simulink model "exp6"  (R2025b)
settings: Solver=VariableStepAuto  StartTime=0.0  StopTime=10.0  RelTol=1e-3
settings Model: Creator=SUBHASH  LastModifiedBy=SUBHASH

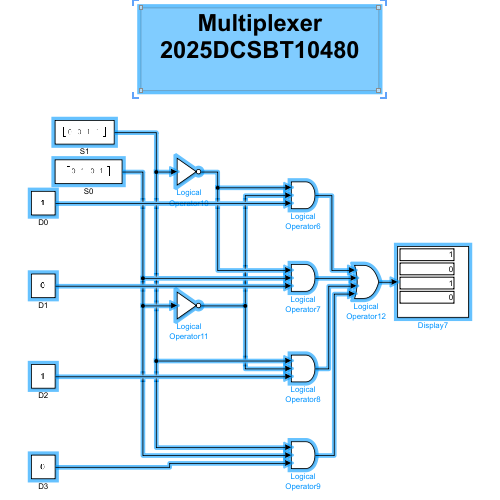
[thumbnail: Simulink's stored preview of the top-level diagram]
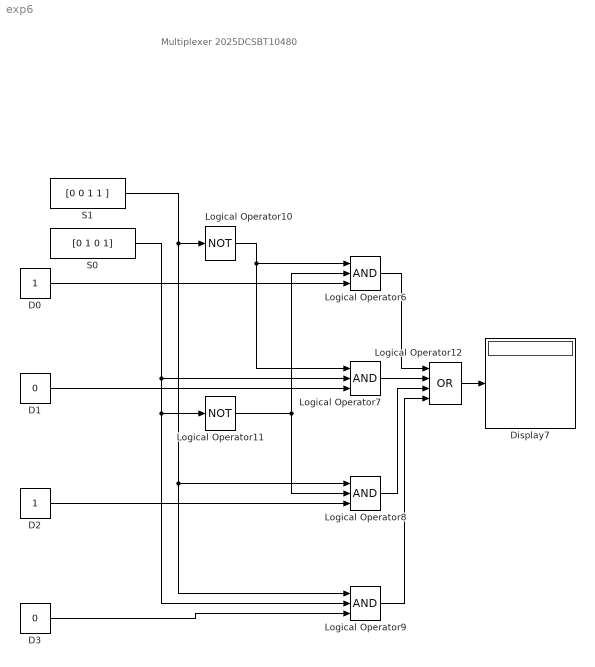
== system exp6 ==
  note: Multiplexer
      | 2025DCSBT10480
  D0 : Constant
  D1 : Constant  Value=0
  D2 : Constant
  D3 : Constant  Value=0
  Display7 : Display
  Logical Operator10 : Logic  Operator=NOT  IconShape=distinctive  AllPortsSameDT=off  OutDataTypeStr=boolean
  Logical Operator11 : Logic  Operator=NOT  IconShape=distinctive  AllPortsSameDT=off  OutDataTypeStr=boolean
  Logical Operator12 : Logic  Operator=OR  Inputs=4  IconShape=distinctive  AllPortsSameDT=off  OutDataTypeStr=boolean
  Logical Operator{6..9} (4 alike) : Logic  Inputs=3  IconShape=distinctive  AllPortsSameDT=off  OutDataTypeStr=boolean
  S0 : Constant  Value=[0 1 0 1]
  S1 : Constant  Value=[0 0 1 1 ]
  wires:
  D2/1 -> Logical Operator8/3
  D0/1 -> Logical Operator6/3
  Logical Operator10/1 -> Logical Operator7/1, Logical Operator6/1
  Logical Operator12/1 -> Display7/1
  Logical Operator11/1 -> Logical Operator8/2, Logical Operator6/2
  S0/1 -> Logical Operator9/2, Logical Operator11/1, Logical Operator7/2
  D1/1 -> Logical Operator7/3
  Logical Operator8/1 -> Logical Operator12/3
  Logical Operator9/1 -> Logical Operator12/4
  Logical Operator7/1 -> Logical Operator12/2
  D3/1 -> Logical Operator9/3
  Logical Operator6/1 -> Logical Operator12/1
  S1/1 -> Logical Operator9/1, Logical Operator8/1, Logical Operator10/1
